simulink model "Unity_NUnityFeed"  (R2019b)
settings: Solver=VariableStepAuto  StartTime=0.0  StopTime=10.0  RelTol=1e-3
libraries: simulink_extras x3
settings Model: Creator=Shishir  LastModifiedBy=Shishir

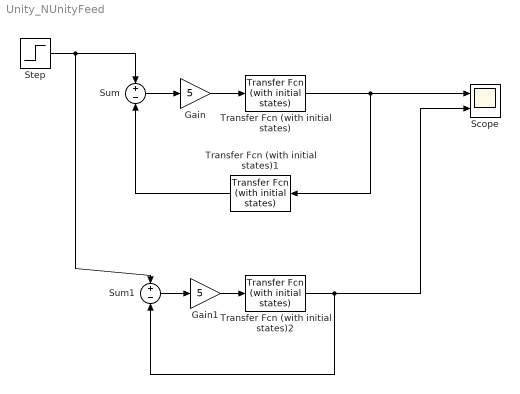
== system Unity_NUnityFeed ==
  Gain : Gain  Gain=5
  Gain1 : Gain  Gain=5
  Scope : Scope  NumInputPorts=2
  Step : Step  Time=0  SampleTime=0
  Sum : Sum  Inputs=+-
  Sum1 : Sum  Inputs=+-
  Transfer Fcn (with initial states) : simulink_extras/Additional Linear/Transfer Fcn (with initial states)  N=[1]  D="[1  1]"  X0=0
  Transfer Fcn (with initial states)1 : simulink_extras/Additional Linear/Transfer Fcn (with initial states)  N=[1]  D="[1  2]"  X0=0
  Transfer Fcn (with initial states)2 : simulink_extras/Additional Linear/Transfer Fcn (with initial states)  N=[1 2]  D="[1  2 1]"  X0=0
  wires:
  Transfer Fcn (with initial states)/1 -> Transfer Fcn (with initial states)1/1, Scope/1
  Transfer Fcn (with initial states)1/1 -> Sum/2
  Gain/1 -> Transfer Fcn (with initial states)/1
  Sum/1 -> Gain/1
  Step/1 -> Sum/1, Sum1/1
  Transfer Fcn (with initial states)2/1 -> Sum1/2, Scope/2
  Sum1/1 -> Gain1/1
  Gain1/1 -> Transfer Fcn (with initial states)2/1
